simulink model "RizzoModel"  (Simulink 7.5)
settings: Solver=ode23tb  StartTime=0.0  StopTime=0.5  RelTol=1e-3
values from neighbouring files (symbols this model uses):
  B1 = 0    [B1P3_Torsonal_Model_1_Coupler_Constants.m]    (also in B1P6_Torsonal_Model_2_Coupler_Constants.m; Torsonal_Model_Constants.m)
  Bc = 0.01    [B1P3_Torsonal_Model_1_Coupler_Constants.m]    (also in Torsonal_Model_Constants.m)
  BL = 0    [B1P3_Torsonal_Model_1_Coupler_Constants.m]    (also in Torsonal_Model_Constants.m)
  J1 = 0.0033    [B1P3_Torsonal_Model_1_Coupler_Constants.m]    (also in B1P6_Torsonal_Model_2_Coupler_Constants.m = 0.0023; Torsonal_Model_Constants.m = 0.0023)
  JL = 0.0033    [B1P15_Torsonal_Model_From_V_Rizzo_One_Coupler_Constants.m]    (also in B1P3_Torsonal_Model_1_Coupler_Constants.m = 0.0023; RizzoConst.m; Torsonal_Model_Constants.m)
  K = 1000    [B1P3_Torsonal_Model_1_Coupler_Constants.m]    (also in Torsonal_Model_Constants.m = 55)
  Ka = 10    [B1P15_Torsonal_Model_From_V_Rizzo_One_Coupler_Constants.m]    (also in RizzoConst.m)
  Ke = 10    [B1P15_Torsonal_Model_From_V_Rizzo_One_Coupler_Constants.m]    (also in RizzoConst.m)
  Kt = 10    [B1P15_Torsonal_Model_From_V_Rizzo_One_Coupler_Constants.m]    (also in RizzoConst.m)
  R = 10    [B1P15_Torsonal_Model_From_V_Rizzo_One_Coupler_Constants.m]    (also in RizzoConst.m)
settings Model: Creator=geovana  LastModifiedBy=geovana
settings OptimizationCC: InitFltsAndDblsToZero=on
settings DebuggingCC: SaveWithParameterizedLinksMsg=none  SignalResolutionControl=TryResolveAllWithWarning  MultiTaskDSMMsg=warning  MultiTaskCondExecSysMsg=none  StrictBusMsg=Warning
settings RTWCC: IncludeERTFirstTime=on
settings GRTTargetCC: TargetFcnLib=ansi_tfl_tmw.mat

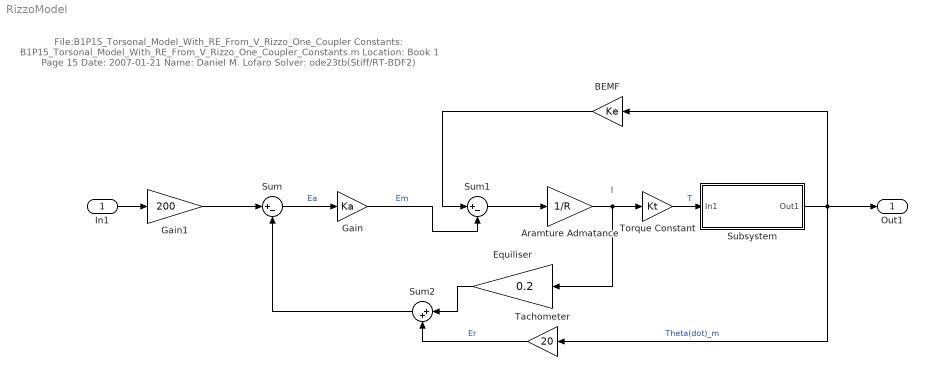
== system RizzoModel ==
  note: File:B1P15_Torsonal_Model_With_RE_From_V_Rizzo_One_Coupler
      | Constants: B1P15_Torsonal_Model_With_RE_From_V_Rizzo_One_Coupler_Constants.m
      | Location: Book 1 Page 15
      | Date: 2007-01-21
      | Name: Daniel M. Lofaro
      | Solver: ode23tb(Stiff/RT-BDF2)
  note: I
  In1 : Inport  OutDataType=fixdt(1, 16)  OutScaling=2^0
  Aramture Admatance : Gain  Gain=1/R  ParameterDataType=sfix(16)  ParameterScaling=2^0  OutDataType=sfix(16)  OutScaling=2^0
  BEMF : Gain  Gain=Ke  ParameterDataType=sfix(16)  ParameterScaling=2^0  OutDataType=sfix(16)  OutScaling=2^0
  Equiliser : Gain  Gain=0.2  ParameterDataType=sfix(16)  ParameterScaling=2^0  OutDataType=sfix(16)  OutScaling=2^0
  Gain : Gain  Gain=Ka  ParameterDataType=sfix(16)  ParameterScaling=2^0  OutDataType=sfix(16)  OutScaling=2^0
  Gain1 : Gain  Gain=200  ParameterDataType=sfix(16)  ParameterScaling=2^0  OutDataType=sfix(16)  OutScaling=2^0
  Subsystem : Subsystem
  Sum : Sum  Inputs=|+-  OutDataType=sfix(16)  OutScaling=2^0
  Sum1 : Sum  Inputs=|+-  OutDataType=sfix(16)  OutScaling=2^0
  Sum2 : Sum  Inputs=|++  OutDataType=sfix(16)  OutScaling=2^0
  Tachometer : Gain  Gain=20  ParameterDataType=sfix(16)  ParameterScaling=2^0  OutDataType=sfix(16)  OutScaling=2^0
  Torque Constant : Gain  Gain=Kt  ParameterDataType=sfix(16)  ParameterScaling=2^0  OutDataType=sfix(16)  OutScaling=2^0
  Out1 : Outport  OutDataType=sfix(16)  OutScaling=2^0
  wires:
  Sum/1 -> Gain/1  "Ea"
  Sum1/1 -> Aramture Admatance/1
  Aramture Admatance/1 -> Torque Constant/1, Equiliser/1
  Torque Constant/1 -> Subsystem/1(In1)  "T"
  BEMF/1 -> Sum1/1
  Gain/1 -> Sum1/2  "Em"
  Subsystem/1(Out1) -> Out1/1, BEMF/1, Tachometer/1  "Theta(dot)_m"
  Tachometer/1 -> Sum2/2  "Er"
  Sum2/1 -> Sum/2
  Equiliser/1 -> Sum2/1
  In1/1 -> Gain1/1
  Gain1/1 -> Sum/1

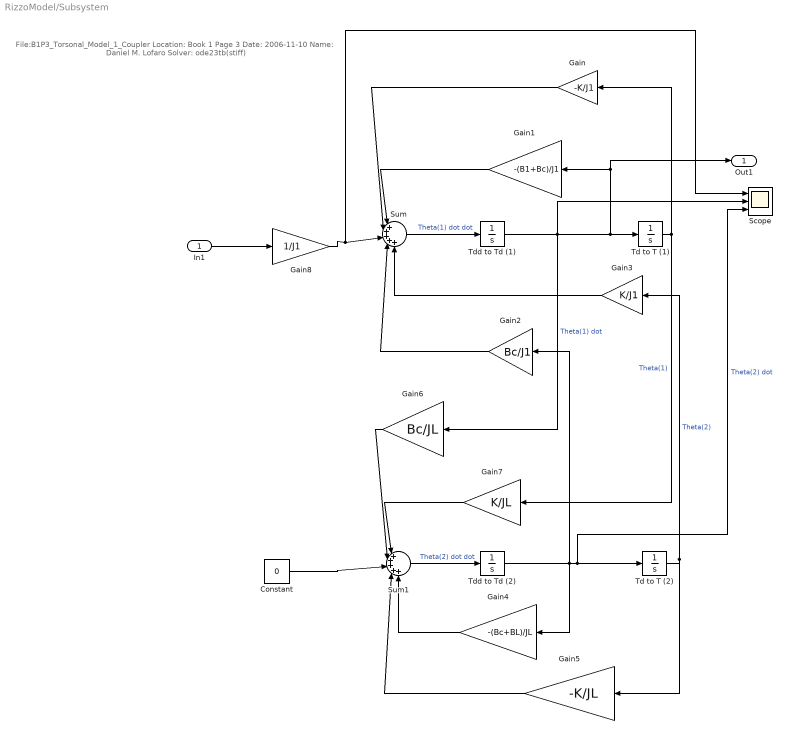
== system RizzoModel/Subsystem ==
  note: File:B1P3_Torsonal_Model_1_Coupler
      | Location: Book 1 Page 3
      | Date: 2006-11-10
      | Name: Daniel M. Lofaro
      | Solver: ode23tb(stiff)
  In1 : Inport  OutDataType=fixdt(1, 16)  OutScaling=2^0
  Constant : Constant  Value=0  OutDataType=sfix(16)  OutScaling=2^0
  Gain : Gain  Gain=-K/J1  ParameterDataType=sfix(16)  ParameterScaling=2^0  OutDataType=sfix(16)  OutScaling=2^0
  Gain1 : Gain  Gain=-(B1+Bc)/J1  ParameterDataType=sfix(16)  ParameterScaling=2^0  OutDataType=sfix(16)  OutScaling=2^0
  Gain2 : Gain  Gain=Bc/J1  ParameterDataType=sfix(16)  ParameterScaling=2^0  OutDataType=sfix(16)  OutScaling=2^0
  Gain3 : Gain  Gain=K/J1  ParameterDataType=sfix(16)  ParameterScaling=2^0  OutDataType=sfix(16)  OutScaling=2^0
  Gain4 : Gain  Gain=-(Bc+BL)/JL  ParameterDataType=sfix(16)  ParameterScaling=2^0  OutDataType=sfix(16)  OutScaling=2^0
  Gain5 : Gain  Gain=-K/JL  ParameterDataType=sfix(16)  ParameterScaling=2^0  OutDataType=sfix(16)  OutScaling=2^0
  Gain6 : Gain  Gain=Bc/JL  ParameterDataType=sfix(16)  ParameterScaling=2^0  OutDataType=sfix(16)  OutScaling=2^0
  Gain7 : Gain  Gain=K/JL  ParameterDataType=sfix(16)  ParameterScaling=2^0  OutDataType=sfix(16)  OutScaling=2^0
  Gain8 : Gain  Gain=1/J1  ParameterDataType=sfix(16)  ParameterScaling=2^0  OutDataType=sfix(16)  OutScaling=2^0
  Scope : Scope  NumInputPorts=3
      settings: YMin=-5~-5~-5  YMax=5~5~5  MaxDataPoints=50000
  Sum : Sum  Inputs=|+++++  OutDataType=sfix(16)  OutScaling=2^0
  Sum1 : Sum  Inputs=|+++++  OutDataType=sfix(16)  OutScaling=2^0
  Td to T (1) : Integrator
  Td to T (2) : Integrator
  Tdd to Td (1) : Integrator
  Tdd to Td (2) : Integrator
  Out1 : Outport  OutDataType=fixdt(1, 16)  OutScaling=2^0
  wires:
  Tdd to Td (2)/1 -> Gain2/1, Gain4/1, Td to T (2)/1, Scope/3  "Theta(2) dot"
  Tdd to Td (1)/1 -> Gain6/1, Td to T (1)/1, Gain1/1, Out1/1, Scope/2  "Theta(1) dot"
  Td to T (1)/1 -> Gain7/1, Gain/1  "Theta(1)"
  Sum/1 -> Tdd to Td (1)/1  "Theta(1) dot dot"
  Gain/1 -> Sum/2
  Gain1/1 -> Sum/1
  Sum1/1 -> Tdd to Td (2)/1  "Theta(2) dot dot"
  Gain2/1 -> Sum/4
  Gain3/1 -> Sum/5
  Td to T (2)/1 -> Gain5/1, Gain3/1  "Theta(2)"
  Gain4/1 -> Sum1/5
  Gain5/1 -> Sum1/4
  Gain6/1 -> Sum1/2
  Gain7/1 -> Sum1/1
  Constant/1 -> Sum1/3
  Gain8/1 -> Sum/3, Scope/1
  In1/1 -> Gain8/1
